simulink model "Sim_localization_1_3"  (R2025b)
settings: Solver=VariableStepAuto  StartTime=0.0  StopTime=T_SIM  MaxStep=0.001  RelTol=1e-3
values from neighbouring files (symbols this model uses):
  d = 0.165    [EX_opt_1.m]    (also in id_LEO.m; init_localization.m; init_localization_template.m; script_init_localization.m)
  D = diag([0.001, 0.001, 0.0175/6, 0.0175/6, 0.0175/6, 0.0175/6*T_s, 0.0175/6*T_s].^2)    [EX_opt_1.m]    (also in init_localization.m; init_localization_template.m; script_init_localization.m)
  d_actual = 0.164    [EX_opt_1.m]    (also in data_for_identification.mat = 0.165; init_localization.m; init_localization_template.m; script_init_localization.m)
  P_INIT_EKF = diag([0.001, 0.001, 0.0175/6, 0.0175/6, 0.0175/6, 0.0175/6*T_s, 0.0175/6*T_s].^2)    [EX_opt_1.m]    (also in init_localization.m; init_localization_template.m; script_init_localization.m)
  PHI_INIT = [0;0]    [EX_opt_1.m]    (also in data_for_identification.mat = [0 0]; id_LEO.m; init_localization.m; init_localization_template.m)
  Q_INIT = q(:,1)    [EX_opt_1.m]    (also in data_for_identification.mat = [0 0 0.463647609001]; id_LEO.m; init_localization.m = [0;0;0]; script_init_localization.m)
  Q_INIT_LOC = Q_INIT    [EX_opt_1.m]    (also in init_localization.m = [0;0;0]; script_init_localization.m = Q_INIT + [0.2; 0.2; deg2rad(15)])
  r = 0.03    [EX_opt_1.m]    (also in id_LEO.m; init_localization.m; init_localization_template.m; script_init_localization.m)
  R_2 = diag([ENCODER_QUANTIZATION/6, ENCODER_QUANTIZATION/6].^2)    [EX_opt_1.m]    (also in init_localization.m = diag([ENCODER_QUANRIZATION/6,ENCODER_QUANRIZATION/6].^2); init_localization_template.m = diag([ENCODER_QUANRIZATION/6,ENCODER_QUANRIZATION/6].^2); script_init_localization.m = diag([ENCODER_QUANRIZATION/6,ENCODER_QUANRIZATION/6].^2))
  R_4 = diag([noise_std, noise_std, ENCODER_QUANTIZATION/6, ENCODER_QUANTIZATION/6].^2)    [EX_opt_1.m]    (also in init_localization.m = diag(([0.001, 0.001, ENCODER_QUANRIZATION/6,ENCODER_QUANRIZA; init_localization_template.m = diag(([0.001, 0.001, ENCODER_QUANRIZATION/6,ENCODER_QUANRIZA; script_init_localization.m = diag(([0.001, 0.001, ENCODER_QUANRIZATION/6,ENCODER_QUANRIZA)
  r_actual = 0.031    [EX_opt_1.m]    (also in data_for_identification.mat = 0.03; init_localization.m; init_localization_template.m; script_init_localization.m)
  T_s = 0.04    [EX_opt_1.m]    (also in EX_opt_2.m = Ts_values(i); data_for_identification.mat; id_LEO.m; id_template.m)
  Z_INIT_EKF = [Q_INIT_LOC; 0; 0; 0; 0]    [EX_opt_1.m]    (also in init_localization.m = [0;0;0])
settings Model: Creator=alberto  LastModifiedBy=loren
settings RTWCC: GPUComputeCapability=3.5

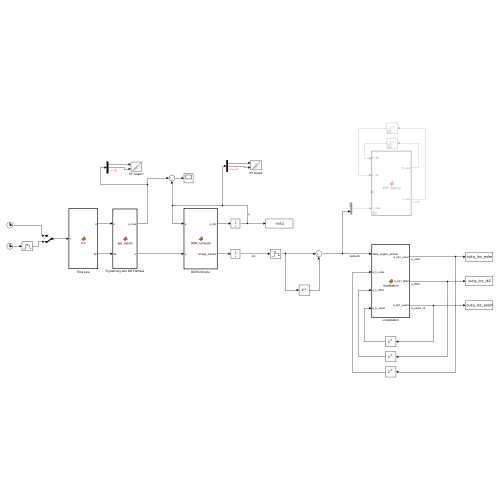
[thumbnail: Simulink's stored preview of the top-level diagram]
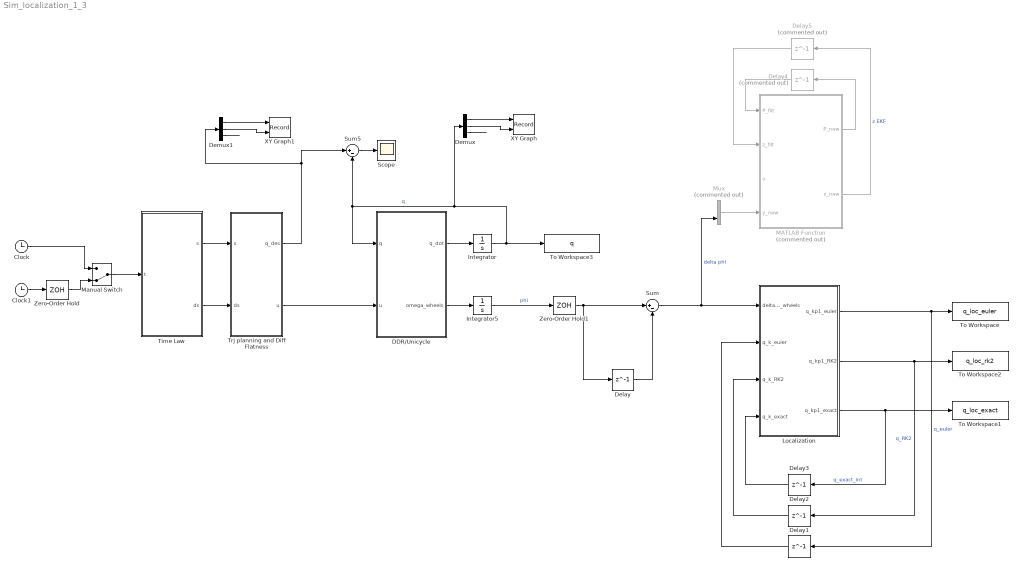
== system Sim_localization_1_3 ==
  Clock : Clock
  Clock1 : Clock
  DDR/Unicycle : MATLAB Function  TreatAsAtomicUnit=on
  Delay : Delay  DelayLength=1  InitialCondition=[0;0]  SampleTime=T_s
  Delay1 : Delay  DelayLength=1  InitialCondition=Q_INIT_LOC
  Delay2 : Delay  DelayLength=1  InitialCondition=Q_INIT_LOC
  Delay3 : Delay  DelayLength=1  InitialCondition=Q_INIT_LOC
  Delay4 : Delay  Commented=on  DelayLength=1  InitialCondition=P_INIT_EKF  SampleTime=T_s
  Delay5 : Delay  Commented=on  DelayLength=1  InitialCondition=Z_INIT_EKF  SampleTime=T_s
  Demux : Demux  Outputs=3
  Demux1 : Demux  Outputs=3
  Integrator : Integrator  InitialCondition=Q_INIT
  Integrator5 : Integrator  InitialCondition=PHI_INIT
  Localization : MATLAB Function  TreatAsAtomicUnit=on
  MATLAB Function : MATLAB Function  Commented=on  TreatAsAtomicUnit=on
  Manual Switch : ManualSwitch  CurrentSetting=0
  Mux : Mux  Commented=on  Inputs=2
  Scope : Scope
      settings: ActiveDisplayYMinimum=-0.088238983771591131  ActiveDisplayYMaximum=0.051968081905583233
  Sum : Sum  Inputs=|+-
  Sum5 : Sum  Inputs=|+-
  Time Law : MATLAB Function  TreatAsAtomicUnit=on
  To Workspace : ToWorkspace  VariableName=q_loc_euler  SaveFormat=Structure With Time  SampleTime=-1
  To Workspace1 : ToWorkspace  VariableName=q_loc_exact  SaveFormat=Structure With Time  SampleTime=-1
  To Workspace2 : ToWorkspace  VariableName=q_loc_rk2  SaveFormat=Structure With Time  SampleTime=-1
  To Workspace3 : ToWorkspace  VariableName=q  SaveFormat=Structure With Time  SampleTime=-1
  Trj planning and Diff Flatness : MATLAB Function  TreatAsAtomicUnit=on
  XY Graph : Record  NumPorts=2.0  FileSettingsInternal="{\"entries\":[{\"content\":{\"excelSettings\":{\"content\":{},\"type\":\"Streamout.ExcelSettings\"},\"parquetSettings\":{\"content\":{},\"type\":\"Streamout.ParquetSettings\"}},\"type\":\"Streamout.FileSettingStorage\",\"uuid\":\"\"}],\"packageUris\":[\"http:\\/\\/schema.mathworks.com\\/mf0\\/streamout_blocks\\/R2020a\"],\"version\":\"1.0\"}"  FrameSettings=[0, 0]  Layout=[1 1]  SignalsInternal="{\"entries\":[{\"content\":{\"signals\":[{\"content\":{\"blockPath\":[],\"dimensions\":[1,1],\"domain\":\"\",\"lineColor\":\"#a2142f\",\"plots\":[ 1 ],\"port\":1,\"signalID\":1,\"signalName\":\"Demux:1\"},\"type\":\"RecordBlkView.Signal\",\"uuid\":\"\"},{\"content\":{\"blockPath\":[],\"dimensions\":[1,1],\"domain\":\"\",\"lineColor\":\"#139fff\",\"plots\":[ 1 ],\"port\":2,\"signalID\":2,\"signalName\":\"Demux:2\"},\"type\":\"RecordBlkView.Signal\",\"uuid\":\"\"}]},\"type\":\"RecordBlkView.InputSignals\",\"uuid\":\"\"}],\"packageUris\":[\"http:\\/\\/schema.mathworks.com\\/mf0\\/streamout_blocks\\/R2020a\"],\"version\":\"1.0\"}"  VisualizationBindings="{\"xyplotplugin\":{\"info\":[{\"series\":[{\"bindingParametersList\":[{\"parameter\":\"X-Axis\",\"signalID\":1,\"signalName\":\"Demux:1\"},{\"parameter\":\"Y-Axis\",\"signalID\":2,\"signalName\":\"Demux:2\"}],\"seriesID\":0}],\"subplotID\":1}]}}"  CompatibilityTag=XY
  XY Graph1 : Record  NumPorts=2.0  FileSettingsInternal="{\"entries\":[{\"content\":{\"excelSettings\":{\"content\":{},\"type\":\"Streamout.ExcelSettings\"},\"parquetSettings\":{\"content\":{},\"type\":\"Streamout.ParquetSettings\"}},\"type\":\"Streamout.FileSettingStorage\",\"uuid\":\"\"}],\"packageUris\":[\"http:\\/\\/schema.mathworks.com\\/mf0\\/streamout_blocks\\/R2020a\"],\"version\":\"1.0\"}"  FrameSettings=[0, 0]  Layout=[1 1]  SignalsInternal="{\"entries\":[{\"content\":{\"signals\":[{\"content\":{\"blockPath\":[],\"dimensions\":[1,1],\"domain\":\"\",\"lineColor\":\"#a2142f\",\"plots\":[ 1 ],\"port\":1,\"signalID\":1,\"signalName\":\"Demux1:1\"},\"type\":\"RecordBlkView.Signal\",\"uuid\":\"\"},{\"content\":{\"blockPath\":[],\"dimensions\":[1,1],\"domain\":\"\",\"lineColor\":\"#139fff\",\"plots\":[ 1 ],\"port\":2,\"signalID\":2,\"signalName\":\"Demux1:2\"},\"type\":\"RecordBlkView.Signal\",\"uuid\":\"\"}]},\"type\":\"RecordBlkView.InputSignals\",\"uuid\":\"\"}],\"packageUris\":[\"http:\\/\\/schema.mathworks.com\\/mf0\\/streamout_blocks\\/R2020a\"],\"version\":\"1.0\"}"  VisualizationBindings="{\"xyplotplugin\":{\"info\":[{\"series\":[{\"bindingParametersList\":[{\"parameter\":\"X-Axis\",\"signalID\":1,\"signalName\":\"Demux1:1\"},{\"parameter\":\"Y-Axis\",\"signalID\":2,\"signalName\":\"Demux1:2\"}],\"seriesID\":0}],\"subplotID\":1}]}}"  CompatibilityTag=XY
  Zero-Order Hold : ZeroOrderHold  SampleTime=T_s
  Zero-Order Hold1 : ZeroOrderHold  SampleTime=T_s
  wires:
  Clock/1 -> Manual Switch/1
  Trj planning and Diff Flatness/2(u) -> DDR/Unicycle/2(u)
  Zero-Order Hold1/1 -> Sum/1, Delay/1
  Delay/1 -> Sum/2
  Delay1/1 -> Localization/2(q_k_euler)
  Sum/1 -> Mux/2, Localization/1(delta_angles_wheels)  "delta phi"
  Integrator/1 -> Demux/1, Sum5/2, DDR/Unicycle/1(q), To Workspace3/1  "q"
  Delay3/1 -> Localization/4(q_k_exact)
  Delay2/1 -> Localization/3(q_k_RK2)
  Localization/2(q_kp1_RK2) -> To Workspace2/1, Delay2/1  "q_RK2"
  Localization/3(q_kp1_exact) -> To Workspace1/1, Delay3/1  "q_exact_int"
  Time Law/1(s) -> Trj planning and Diff Flatness/1(s)
  Time Law/2(ds) -> Trj planning and Diff Flatness/2(ds)
  DDR/Unicycle/1(q_dot) -> Integrator/1
  Sum5/1 -> Scope/1
  Integrator5/1 -> Zero-Order Hold1/1  "phi"
  MATLAB Function/1(P_new) -> Delay4/1
  Delay4/1 -> MATLAB Function/1(P_filt)
  Delay5/1 -> MATLAB Function/2(z_filt)
  MATLAB Function/2(z_new) -> Delay5/1  "z EKF"
  Mux/1 -> MATLAB Function/4(y_new)
  Demux/1 -> XY Graph/1
  Demux/3 -> ?
  Demux/2 -> XY Graph/2
  Trj planning and Diff Flatness/1(q_des) -> Sum5/1, Demux1/1
  Demux1/2 -> XY Graph1/2
  Demux1/1 -> XY Graph1/1
  Demux1/3 -> ?
  Manual Switch/1 -> Time Law/1(t)
  Zero-Order Hold/1 -> Manual Switch/2
  Clock1/1 -> Zero-Order Hold/1
  DDR/Unicycle/2(omega_wheels) -> Integrator5/1
  Localization/1(q_kp1_euler) -> To Workspace/1, Delay1/1  "q_euler"

== matlab function Sim_localization_1_3/Time Law ==
  data: t input; s output; ds output
function [s, ds] = fcn(t)
    
    Ta = 0.5;
    Tc = 9; 
        
    vc = 1/(Ta+Tc);
    a = vc/Ta;
   
    if t < Ta
        s_dot = a*t;
        s = 0.5*a*t^2;
    
    elseif t < (Ta+Tc)
        s_dot = vc;
        s = 0.5*a*Ta^2 + vc*(t - Ta);
    
    elseif t < (2*Ta+Tc)
        s_dot = vc - a*(t - Ta - Tc);
        s = 0.5*a*Ta^2 + vc*Tc + vc*(t - Ta - Tc) ...
            - 0.5*a*(t - Ta - Tc)^2;
    else
        s_dot = 0;
        s = 1;
    end

    ds = s_dot;
    
end

== matlab function Sim_localization_1_3/DDR//Unicycle ==
  data: q input; u input; q_dot output; omega_wheels output; d_actual parameter; r_actual parameter
function [q_dot, omega_wheels] = DDR_Unicycle(q, u, d_actual, r_actual)

    % extract variables
    v = u(1);
    omega = u(2);

    q_dot= zeros(3,1);
    
    q_dot(1) = v*cos(q(3));
    q_dot(2) = v*sin(q(3));
    q_dot(3) = omega;

    
    wL = v/r_actual - d_actual/(2*r_actual) * omega;
    wR = v/r_actual + d_actual/(2*r_actual) * omega;

    omega_wheels = [wL; wR];

end

== matlab function Sim_localization_1_3/Trj planning and Diff Flatness ==
  data: q_des output; s input; u output; ds input
function [q_des, u] = get_inputs(s, ds)

    R = 0.4;
    w = 2*pi;

    % function [x_s, y_s, x_s_dot, y_s_dot, x_s_ddot, y_s_ddot] = gen_eight_shape_trajectory(R, w, s)
   
    x_s = R*sin(2*w*s);
    y_s = R*sin(w*s);
    
    % computes derivatives analytically

    x_s_dot = 2*R*w*cos(2*w*s);
    y_s_dot = R*w*cos(w*s);
    
    x_s_ddot = -4*R*w^2*sin(2*w*s);
    y_s_ddot = -R*w^2*sin(w*s);


    % function [q, u] = flat_to_kinematic_cartesian(x, y, x_dot, y_dot, x_ddot, y_ddot)

    theta = atan2(y_s_dot, x_s_dot);
    
    q_des = [x_s; y_s; theta];
   
    v_tilde = sqrt(x_s_dot^2 + y_s_dot^2);
    omega_tilde = (x_s_dot * y_s_ddot - y_s_dot * x_s_ddot) / (x_s_dot^2 + y_s_dot^2);
    
    % Convert into real Inputs
    v = v_tilde * ds;
    omega = omega_tilde * ds;
    
    u = [v; omega];
end

== matlab function Sim_localization_1_3/Localization ==
  data: delta_angles_wheels input; q_k_euler input; q_k_RK2 input; q_k_exact input; r parameter; d parameter; q_kp1_euler output; T_s parameter; q_kp1_RK2 output; q_kp1_exact output
function [q_kp1_euler, q_kp1_RK2, q_kp1_exact] = localization(delta_angles_wheels, q_k_euler, q_k_RK2, q_k_exact, r, d, T_s)

    % extraction data
    delta_phi_L = delta_angles_wheels(1);
    delta_phi_R = delta_angles_wheels(2);

    x_k_euler = q_k_euler(1); 
    y_k_euler = q_k_euler(2); 
    theta_k_euler = q_k_euler(3);
    
    x_k_RK2 = q_k_RK2(1); 
    y_k_RK2 = q_k_RK2(2); 
    theta_k_RK2 = q_k_RK2(3);

    x_k_exact = q_k_exact(1);
    y_k_exact = q_k_exact(2); 
    theta_k_exact = q_k_exact(3);


    % velocities estimate
    v_k = r / (2*T_s) * (delta_phi_R + delta_phi_L);
    w_k = r / (d*T_s) * (delta_phi_R - delta_phi_L);
    
    % Euler integration
    x_kp1_euler = x_k_euler + v_k * T_s * cos(theta_k_euler);
    y_kp1_euler = y_k_euler + v_k * T_s * sin(theta_k_euler);
    theta_kp1_euler = theta_k_euler + w_k * T_s;
    
    q_kp1_euler = [x_kp1_euler; y_kp1_euler; theta_kp1_euler];
    
    % RK2 Integration
    x_kp1_RK2 = x_k_RK2 + v_k * T_s * cos(theta_k_RK2 + (w_k * T_s)/2);
    y_kp1_RK2 = y_k_RK2 + v_k * T_s * sin(theta_k_RK2 + (w_k * T_s)/2);
    theta_kp1_RK2 = theta_k_RK2 + w_k * T_s;
    
    q_kp1_RK2 = [x_kp1_RK2; y_kp1_RK2; theta_kp1_RK2];
    
    % Exact Integration
    if abs(w_k) < 1e-4
        % use RK2 approximation to avoid division by zero when w_k is near 0
        x_kp1_exact = x_k_exact + v_k * T_s * cos(theta_k_exact + (w_k * T_s)/2);
        y_kp1_exact = y_k_exact + v_k * T_s * sin(theta_k_exact + (w_k * T_s)/2);
    else
        % Exact formulas
        x_kp1_exact = x_k_exact + (v_k / w_k) * (sin(theta_k_exact + w_k * T_s) - sin(theta_k_exact));
        y_kp1_exact = y_k_exact - (v_k / w_k) * (cos(theta_k_exact + w_k * T_s) - cos(theta_k_exact));
    end
    theta_kp1_exact = theta_k_exact + w_k * T_s;
    
    q_kp1_exact = [x_kp1_exact; y_kp1_exact; theta_kp1_exact];
    
end

== matlab function Sim_localization_1_3/MATLAB Function ==
  data: P_filt input; P_new output; z_filt input; z_new output; u input; y_new input; D parameter; R_2 parameter; R_4 parameter; T_s parameter; r parameter; d parameter
function [P_new, z_new] = EKF_filtering(P_filt, z_filt, u, y_new, D, R_2, R_4, T_s, r, d)
